simulink model "Cable_Dynamics_Model_testing"  (R2019b)
settings: Solver=VariableStepAuto  StartTime=0.0  StopTime=10.0  RelTol=1e-3
undefined symbols (not defined in the file or in its folder): a, d, m, p, r, zeta
settings Model: Creator=arund  LastModifiedBy=arund

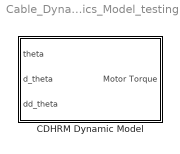
== system Cable_Dynamics_Model_testing ==
  CDHRM Dynamic Model : Subsystem

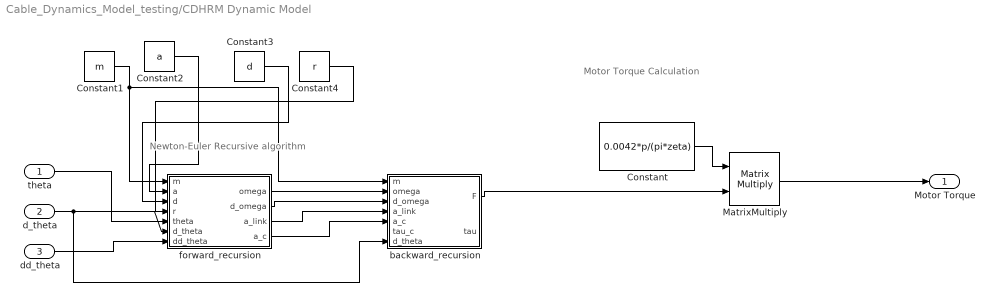
== system Cable_Dynamics_Model_testing/CDHRM Dynamic Model ==
  note: Newton-Euler Recursive algorithm
  note: Motor Torque Calculation
  theta : Inport
  d_theta : Inport  Port=2
  dd_theta : Inport  Port=3
  Constant : Constant  Value=0.0042*p/(pi*zeta)
  Constant1 : Constant  Value=m
  Constant2 : Constant  Value=a
  Constant3 : Constant  Value=d
  Constant4 : Constant  Value=r
  MatrixMultiply : Product  Multiplication=Matrix(*)
  backward_recursion : MATLAB Function  TreatAsAtomicUnit=on
  forward_recursion : MATLAB Function  TreatAsAtomicUnit=on
  Motor Torque : Outport
  wires:
  theta/1 -> forward_recursion/5(theta)
  d_theta/1 -> backward_recursion/7(d_theta), forward_recursion/6(d_theta)
  dd_theta/1 -> forward_recursion/7(dd_theta)
  forward_recursion/1(omega) -> backward_recursion/2(omega)
  forward_recursion/2(d_omega) -> backward_recursion/3(d_omega)
  backward_recursion/1(F) -> MatrixMultiply/2
  MatrixMultiply/1 -> Motor Torque/1
  Constant/1 -> MatrixMultiply/1
  forward_recursion/4(a_c) -> backward_recursion/5(a_c)
  forward_recursion/3(a_link) -> backward_recursion/4(a_link)
  Constant1/1 -> backward_recursion/1(m), forward_recursion/1(m)
  Constant2/1 -> forward_recursion/2(a)
  Constant3/1 -> forward_recursion/3(d)
  Constant4/1 -> forward_recursion/4(r)

== matlab function Cable_Dynamics_Model_testing/CDHRM Dynamic Model/backward_recursion ==
  data: m input; omega input; F output; d_omega input; a_link input; tau output; a_c input; tau_c input; d_theta input
function [F, tau] = fcn(m,omega, d_omega, a_link, a_c,tau_c,d_theta)
N=9;
% Parameters
z_0=[0;0;1];
F_v=0.001;
I=cell(2*N,1);
for i=1:N
    I{2*i-1}=[1/12*(m*(a+2*d)^2)+1/4*(m*r^2) 0 0;
                      0 1/12*(m*(a+2*d)^2)+1/4*(m*r^2) 0;
                      0 0 1/4*(m*r^2)];
    I{2*i}=zeros(3);
end
% Calculate D-H parameter table
DH_params=zeros(2*N,4);
for i=1:N
    if rem(i,2)==0
        DH_params(2*i-1:2*i,:)=[180+(theta(2*i-1)*180/pi) 90 0 0; 180+(theta(2*i)*180/pi) 0 a 0];
    else
        DH_params(2*i-1:2*i,:)=[(theta(2*i-1)*180/pi) 90 0 0; (theta(2*i*180/pi)) 0 a 0];
    end
end

% Calculate transformation matrix n_A_n+1 (A_wrt_prev) and store in cell
% array
R = cell(2*N,1);
for n=1:2*N
    theta_i=DH_params(n,1);
    alpha_i=DH_params(n,2);
    R{n}=[cosd(theta_i) -sind(theta_i)*cosd(alpha_i) sind(theta_i)*sind(alpha_i);...
       sind(theta_i)  cosd(theta_i)*cosd(alpha_i) -cosd(theta_i)*sind(alpha_i);...
                  0              sind(alpha_i)   cosd(alpha_i) ];
end
% Backward Recursion
F=zeros(3,2*N);
mu=zeros(3,2*N);
tau=zeros(3,2*N);
F(:,2*N)=m*a_c(:,2*N);
mu(:,2*N)=-cross()+I{2*N}*d_omega(:,2*N)+cross(omega(:,2*N),I{2*N}*omega(:,2*N));
tau(:,2*N)=mu(:,2*N)*R{2*N}*z_0+tau_c+F_v*d_theta;
for n=2*N-1:-1:1
    F(:,n)=m*a_c(:,n);
    mu(:,n)=-cross()+I{n}*d_omega(:,n)+cross(omega(:,n),I{n}*omega(:,n));
    tau(:,n)=mu(:,n)*R{n}*z_0+tau_c;
end

== matlab function Cable_Dynamics_Model_testing/CDHRM Dynamic Model/forward_recursion ==
  data: m input; a input; d input; r input; theta input; omega output; d_theta input; dd_theta input; d_omega output; a_link output; a_c output
function [omega, d_omega, a_link, a_c] = fcn(m,a,d,r,theta, d_theta, dd_theta)
N=9;
% Parameters
r_c_prev_frame=zeros(3,2*N);
r_c=zeros(3,2*N);
z_0=[0;0;-1];
for i=1:N
    r_c_prev_frame(:,2*i-1:2*i)=[a/2+d 0;...
                            0  0;...
                            0  0];
    r_c(:,2*i-1:2*i)=[-a/2+d 0;...
                        0  0;...
                        0  0];
    r_frames=[a+2*d 0;...
               0    0;...
               0    0];
end
% Calculate D-H parameter table
DH_params=zeros(2*N,4);
for i=1:N
    if rem(i,2)==0
        DH_params(2*i-1:2*i,:)=[180+(theta(2*i-1)*180/pi) 90 0 0; 180+(theta(2*i)*180/pi) 0 a 0];
    else
        DH_params(2*i-1:2*i,:)=[(theta(2*i-1)*180/pi) 90 0 0; (theta(2*i*180/pi)) 0 a 0];
    end
end

% Calculate transformation matrix n_A_n+1 (A_wrt_prev) and store in cell
% array
R = cell(2*N,1);
for n=1:2*N
    theta_i=DH_params(n,1);
    alpha_i=DH_params(n,2);
    R{n}=[cosd(theta_i) -sind(theta_i)*cosd(alpha_i) sind(theta_i)*sind(alpha_i);...
       sind(theta_i)  cosd(theta_i)*cosd(alpha_i) -cosd(theta_i)*sind(alpha_i);...
                  0              sind(alpha_i)   cosd(alpha_i) ];
end
% Forward iteration
% Initialising the matrices
omega=zeros(3,2*N);
d_omega=zeros(3,2*N);
a_link=zeros(3,2*N);
a_c=zeros(3,2*N);

% Calculating link 1 parameters separately
omega(:,1)=R{1}'*d_theta(1)*z_0;
d_omega(:,1)=R{1}'*dd_theta(1)*z_0;
a_link(:,1)=cross(d_omega(:,1),r_frames(:,0))+cross(omega(:,1),cross(omega(:,1),r_frames(:,1)));
a_c(:,1)=a_link(:,1)+cross(d_omega(:,1),r_c(:,1))+cross(omega(:,1),cross(omega(:,1),r_c(:,1)));
for n=2:2*N
    omega(:,n)=R{n}'*(omega(:,n-1)+d_theta(n)*z_0);
    d_omega(:,n)=R{n}'*(d_omega(:,n-1)+dd_theta(n)*z_0+cross(d_theta(n)*omega(:,n-1),z_0));
    a_link=R{n}'*a_link(:,n-1)+cross(d_omega(:,n),r_frames(:,n))+cross(omega(:,n),cross(omega(:,n),r_frames(:,n)));
    a_c=a_link(:,n)+cross(d_omega(:,n),r_c(:,n))+cross(omega(:,n),cross(omega(:,n),r_c(:,n)));
end
